simulink model "Modell_Aufzug"  (Simulink 8.5)
settings: Solver=ode45  StartTime=0.0  StopTime=Inf  MaxStep=step_max  RelTol=1e-3
values from neighbouring files (symbols this model uses):
  CE = 1.528    [Initdatei.m]
  CM = 1.528    [Initdatei.m]
  hsp = 1    [Initdatei.m]
  J = 0.012    [Initdatei.m]
  Kpi = LA/(2*(Tt+Tgl))    (= 1.81818181818)    [Initdatei.m]
  Kpn = (2*pi*J)/(CM*4*(Tt+Tgl))    (= 11.2146334612)    [Initdatei.m]
  Kpx = 1/(2*8*(Tt+Tgl)*hsp)    (= 56.8181818182)    [Initdatei.m]
  MLast = 10    [Initdatei.m]
  RA = 0.250    (= 0.25)    [Initdatei.m]
  TA = LA/RA    (= 0.016)    [Initdatei.m]
  Tgl = 0.001    [Initdatei.m]
  TN = 8*(Tt+Tgl)    (= 0.0088)    [Initdatei.m]
  Tt = 0.0001    [Initdatei.m]
  xSwitch_1_m = 4.50    (= 4.5)    [Initdatei.m]
  xSwitch_1_o = 5.50    (= 5.5)    [Initdatei.m]
  xSwitch_1_u = 3.50    (= 3.5)    [Initdatei.m]
  xSwitch_2_o = 9.0    (= 9)    [Initdatei.m]
  xSwitch_2_u = 8.00    (= 8)    [Initdatei.m]
  xSwitch_EG_o = 1    [Initdatei.m]
  xSwitch_EG_u = 0.20    (= 0.2)    [Initdatei.m]
libraries: simulink x6
settings Model: Creator=Fabian Horst  LastModifiedBy=thomas.stetz
settings DataIOCC: LimitDataPoints=off
settings DebuggingCC: SolverPrmCheckMsg=warning  FcnCallInpInsideContextMsg=UseLocalSettings

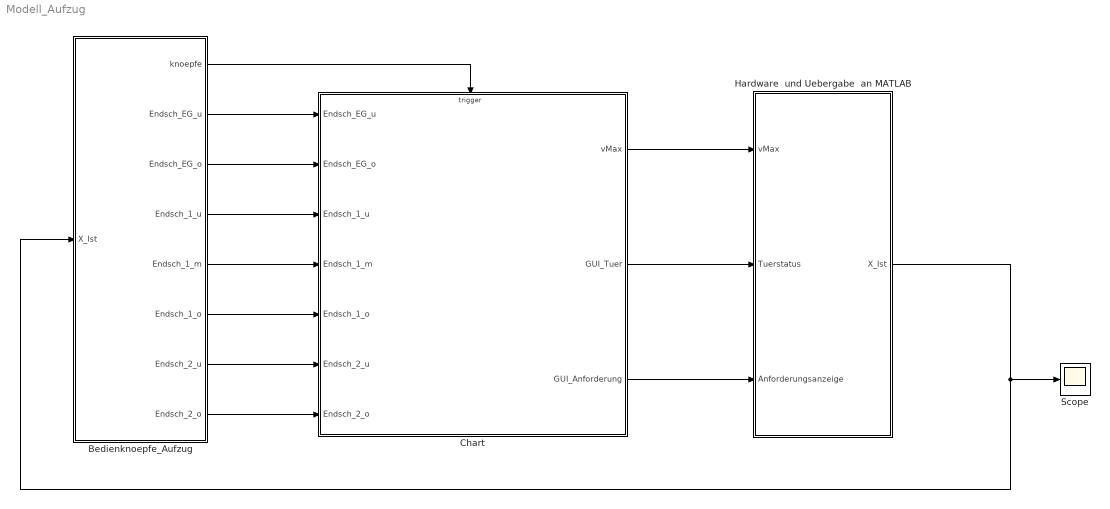
== system Modell_Aufzug ==
  Bedienknoepfe_Aufzug : Subsystem
  Chart : Stateflow chart  TreatAsAtomicUnit=on
  Hardware  und Uebergabe  an MATLAB : Subsystem
  Scope : Scope
  wires:
  Bedienknoepfe_Aufzug/1(knoepfe) -> Chart/Trigger
  Chart/1(vMax) -> Hardware  und Uebergabe  an MATLAB/1(vMax)
  Bedienknoepfe_Aufzug/8(Endsch_2_o) -> Chart/7(Endsch_2_o)
  Bedienknoepfe_Aufzug/2(Endsch_EG_u) -> Chart/1(Endsch_EG_u)
  Bedienknoepfe_Aufzug/3(Endsch_EG_o) -> Chart/2(Endsch_EG_o)
  Bedienknoepfe_Aufzug/4(Endsch_1_u) -> Chart/3(Endsch_1_u)
  Bedienknoepfe_Aufzug/6(Endsch_1_o) -> Chart/5(Endsch_1_o)
  Bedienknoepfe_Aufzug/7(Endsch_2_u) -> Chart/6(Endsch_2_u)
  Chart/2(GUI_Tuer) -> Hardware  und Uebergabe  an MATLAB/2(Tuerstatus)
  Hardware  und Uebergabe  an MATLAB/1(X_Ist) -> Bedienknoepfe_Aufzug/1(X_Ist), Scope/1
  Chart/3(GUI_Anforderung) -> Hardware  und Uebergabe  an MATLAB/3(Anforderungsanzeige)
  Bedienknoepfe_Aufzug/5(Endsch_1_m) -> Chart/4(Endsch_1_m)

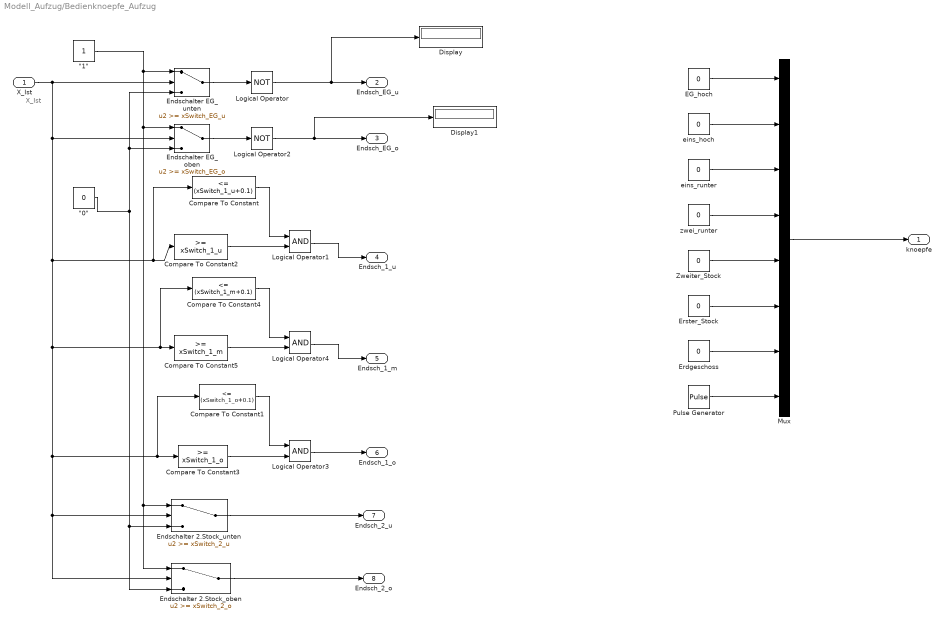
== system Modell_Aufzug/Bedienknoepfe_Aufzug ==
  note: X_Ist
  X_Ist : Inport  Description=X_Ist
  "\"0\"" : Constant  Value=0  OutDataTypeStr=boolean
  "\"1\"" : Constant  OutDataTypeStr=boolean
  Compare To Constant : simulink/Logic and Bit Operations/Compare To Constant  relop=<=  const=(xSwitch_1_u+0.1)  OutDataTypeStr=boolean
  Compare To Constant1 : simulink/Logic and Bit Operations/Compare To Constant  relop=<=  const=(xSwitch_1_o+0.1)  OutDataTypeStr=boolean
  Compare To Constant2 : simulink/Logic and Bit Operations/Compare To Constant  relop=>=  const=xSwitch_1_u  OutDataTypeStr=boolean
  Compare To Constant3 : simulink/Logic and Bit Operations/Compare To Constant  relop=>=  const=xSwitch_1_o  OutDataTypeStr=boolean
  Compare To Constant4 : simulink/Logic and Bit Operations/Compare To Constant  relop=<=  const=(xSwitch_1_m+0.1)  OutDataTypeStr=boolean
  Compare To Constant5 : simulink/Logic and Bit Operations/Compare To Constant  relop=>=  const=xSwitch_1_m  OutDataTypeStr=boolean
  Display : Display
  Display1 : Display
  EG_hoch : Constant  Value=0
  Endschalter 2.Stock_oben : Switch  Threshold=xSwitch_2_o
  Endschalter 2.Stock_unten : Switch  Threshold=xSwitch_2_u
  Endschalter EG_oben : Switch  Threshold=xSwitch_EG_o
  Endschalter EG_unten : Switch  Threshold=xSwitch_EG_u
  Erdgeschoss : Constant  Value=0
  Erster_Stock : Constant  Value=0
  Logical Operator : Logic  Operator=NOT  AllPortsSameDT=off  OutDataTypeStr=boolean
  Logical Operator1 : Logic  AllPortsSameDT=off  OutDataTypeStr=boolean
  Logical Operator2 : Logic  Operator=NOT  AllPortsSameDT=off  OutDataTypeStr=boolean
  Logical Operator3 : Logic  AllPortsSameDT=off  OutDataTypeStr=boolean
  Logical Operator4 : Logic  AllPortsSameDT=off  OutDataTypeStr=boolean
  Mux : Mux  Inputs=8
  Pulse Generator : DiscretePulseGenerator  PulseType=Time based  Period=0.001  PulseWidth=50
  Zweiter_Stock : Constant  Value=0
  eins_hoch : Constant  Value=0
  eins_runter : Constant  Value=0
  zwei_runter : Constant  Value=0
  knoepfe : Outport
  Endsch_EG_u : Outport  Port=2
  Endsch_EG_o : Outport  Port=3
  Endsch_1_u : Outport  Port=4
  Endsch_1_m : Outport  Port=5
  Endsch_1_o : Outport  Port=6
  Endsch_2_u : Outport  Port=7
  Endsch_2_o : Outport  Port=8
  wires:
  EG_hoch/1 -> Mux/1
  eins_hoch/1 -> Mux/2
  eins_runter/1 -> Mux/3
  zwei_runter/1 -> Mux/4
  Zweiter_Stock/1 -> Mux/5
  Erdgeschoss/1 -> Mux/7
  Mux/1 -> knoepfe/1
  "\"1\""/1 -> Endschalter EG_unten/1, Endschalter EG_oben/1, Endschalter 2.Stock_unten/1, Endschalter 2.Stock_oben/1
  "\"0\""/1 -> Endschalter EG_unten/3, Endschalter EG_oben/3, Endschalter 2.Stock_unten/3, Endschalter 2.Stock_oben/3
  X_Ist/1 -> Endschalter EG_unten/2, Compare To Constant/1, Compare To Constant2/1, Compare To Constant1/1, Compare To Constant3/1, Endschalter 2.Stock_oben/2, Endschalter 2.Stock_unten/2, Compare To Constant5/1, Compare To Constant4/1, Endschalter EG_oben/2
  Endschalter 2.Stock_unten/1 -> Endsch_2_u/1
  Erster_Stock/1 -> Mux/6
  Endschalter EG_unten/1 -> Logical Operator/1
  Logical Operator/1 -> Endsch_EG_u/1, Display/1
  Logical Operator1/1 -> Endsch_1_u/1
  Compare To Constant/1 -> Logical Operator1/1
  Compare To Constant2/1 -> Logical Operator1/2
  Pulse Generator/1 -> Mux/8
  Endschalter EG_oben/1 -> Logical Operator2/1
  Logical Operator2/1 -> Endsch_EG_o/1, Display1/1
  Logical Operator3/1 -> Endsch_1_o/1
  Compare To Constant1/1 -> Logical Operator3/1
  Compare To Constant3/1 -> Logical Operator3/2
  Endschalter 2.Stock_oben/1 -> Endsch_2_o/1
  Logical Operator4/1 -> Endsch_1_m/1
  Compare To Constant4/1 -> Logical Operator4/1
  Compare To Constant5/1 -> Logical Operator4/2

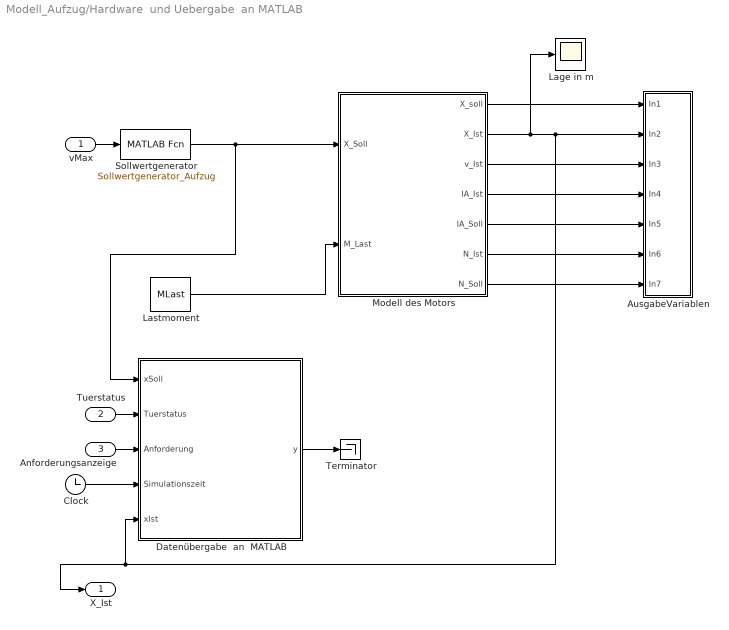
== system Modell_Aufzug/Hardware  und Uebergabe  an MATLAB ==
  vMax : Inport
  Tuerstatus : Inport  Port=2
  Anforderungsanzeige : Inport  Port=3
  AusgabeVariablen : Subsystem
  Clock : Clock
  Datenübergabe  an  MATLAB : MATLAB Function  TreatAsAtomicUnit=on
  Lage in m : Scope
      settings: TimeRange=20  YMin=-1  YMax=14
  Lastmoment : Constant  Value=MLast
  Modell des Motors : Subsystem
  Sollwertgenerator : MATLABFcn  MATLABFcn=Sollwertgenerator_Aufzug
  Terminator : Terminator
  X_Ist : Outport
  wires:
  Modell des Motors/1(X_soll) -> AusgabeVariablen/1(In1)
  Modell des Motors/2(X_Ist) -> AusgabeVariablen/2(In2), Datenübergabe  an  MATLAB/5(xIst), X_Ist/1, Lage in m/1
  Modell des Motors/3(v_Ist) -> AusgabeVariablen/3(In3)
  Modell des Motors/4(IA_Ist) -> AusgabeVariablen/4(In4)
  Modell des Motors/5(IA_Soll) -> AusgabeVariablen/5(In5)
  Modell des Motors/6(N_Ist) -> AusgabeVariablen/6(In6)
  Modell des Motors/7(N_Soll) -> AusgabeVariablen/7(In7)
  Lastmoment/1 -> Modell des Motors/2(M_Last)
  Clock/1 -> Datenübergabe  an  MATLAB/4(Simulationszeit)
  Sollwertgenerator/1 -> Datenübergabe  an  MATLAB/1(xSoll), Modell des Motors/1(X_Soll)
  vMax/1 -> Sollwertgenerator/1
  Tuerstatus/1 -> Datenübergabe  an  MATLAB/2(Tuerstatus)
  Datenübergabe  an  MATLAB/1(y) -> Terminator/1
  Anforderungsanzeige/1 -> Datenübergabe  an  MATLAB/3(Anforderung)

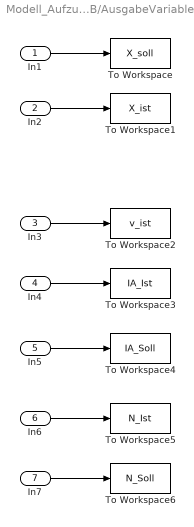
== system Modell_Aufzug/Hardware  und Uebergabe  an MATLAB/AusgabeVariablen ==
  In1 : Inport
  In2 : Inport  Port=2
  In3 : Inport  Port=3
  In4 : Inport  Port=4
  In5 : Inport  Port=5
  In6 : Inport  Port=6
  In7 : Inport  Port=7
  To Workspace : ToWorkspace  VariableName=X_soll  SaveFormat=Structure  SampleTime=-1
  To Workspace1 : ToWorkspace  VariableName=X_ist  SaveFormat=Structure  SampleTime=-1
  To Workspace2 : ToWorkspace  VariableName=v_ist  SaveFormat=Structure  SampleTime=-1
  To Workspace3 : ToWorkspace  VariableName=IA_Ist  SaveFormat=Structure  SampleTime=-1
  To Workspace4 : ToWorkspace  VariableName=IA_Soll  SaveFormat=Structure  SampleTime=-1
  To Workspace5 : ToWorkspace  VariableName=N_Ist  SaveFormat=Structure  SampleTime=-1
  To Workspace6 : ToWorkspace  VariableName=N_Soll  SaveFormat=Structure  SampleTime=-1
  wires:
  In1/1 -> To Workspace/1
  In2/1 -> To Workspace1/1
  In3/1 -> To Workspace2/1
  In4/1 -> To Workspace3/1
  In5/1 -> To Workspace4/1
  In6/1 -> To Workspace5/1
  In7/1 -> To Workspace6/1

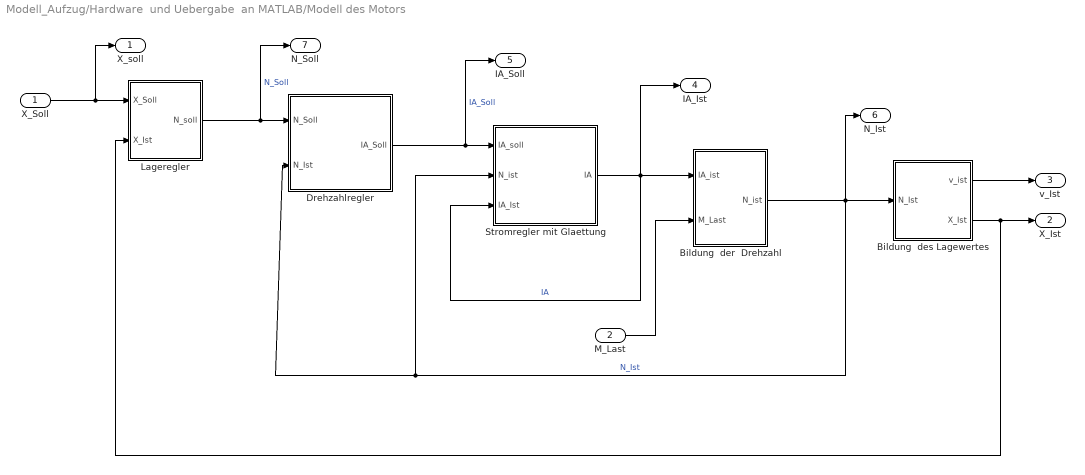
== system Modell_Aufzug/Hardware  und Uebergabe  an MATLAB/Modell des Motors ==
  X_Soll : Inport
  M_Last : Inport  Port=2
  Bildung  der  Drehzahl : Subsystem
  Bildung  des Lagewertes : Subsystem
  Drehzahlregler : Subsystem
  Lageregler : Subsystem
  Stromregler mit Glaettung : Subsystem
  X_soll : Outport
  X_Ist : Outport  Port=2
  v_Ist : Outport  Port=3
  IA_Ist : Outport  Port=4
  IA_Soll : Outport  Port=5
  N_Ist : Outport  Port=6
  N_Soll : Outport  Port=7
  wires:
  Lageregler/1(N_soll) -> Drehzahlregler/1(N_Soll), N_Soll/1  "N_Soll"
  Drehzahlregler/1(IA_Soll) -> Stromregler mit Glaettung/1(IA_soll), IA_Soll/1  "IA_Soll"
  X_Soll/1 -> Lageregler/1(X_Soll), X_soll/1
  Stromregler mit Glaettung/1(IA) -> Bildung  der  Drehzahl/1(IA_ist), Stromregler mit Glaettung/3(IA_Ist), IA_Ist/1  "IA"
  Bildung  der  Drehzahl/1(N_ist) -> Bildung  des Lagewertes/1(N_Ist), Drehzahlregler/2(N_Ist), Stromregler mit Glaettung/2(N_ist), N_Ist/1  "N_Ist"
  M_Last/1 -> Bildung  der  Drehzahl/2(M_Last)
  Bildung  des Lagewertes/1(v_ist) -> v_Ist/1
  Bildung  des Lagewertes/2(X_Ist) -> X_Ist/1, Lageregler/2(X_Ist)

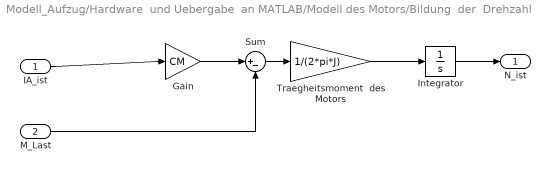
== system Modell_Aufzug/Hardware  und Uebergabe  an MATLAB/Modell des Motors/Bildung  der  Drehzahl ==
  IA_ist : Inport
  M_Last : Inport  Port=2
  Gain : Gain  Gain=CM
  Integrator : Integrator
  Sum : Sum  Inputs=|+-
  Traegheitsmoment  des Motors : Gain  Gain=1/(2*pi*J)
  N_ist : Outport
  wires:
  IA_ist/1 -> Gain/1
  M_Last/1 -> Sum/2
  Gain/1 -> Sum/1
  Sum/1 -> Traegheitsmoment  des Motors/1
  Traegheitsmoment  des Motors/1 -> Integrator/1
  Integrator/1 -> N_ist/1

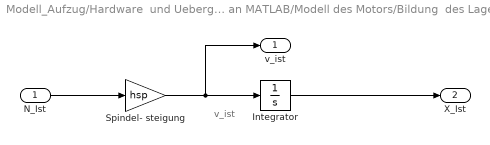
== system Modell_Aufzug/Hardware  und Uebergabe  an MATLAB/Modell des Motors/Bildung  des Lagewertes ==
  note: v_ist
  N_Ist : Inport
  Integrator : Integrator
  Spindel- steigung : Gain  Gain=hsp
  v_ist : Outport
  X_Ist : Outport  Port=2
  wires:
  N_Ist/1 -> Spindel- steigung/1
  Spindel- steigung/1 -> Integrator/1, v_ist/1
  Integrator/1 -> X_Ist/1

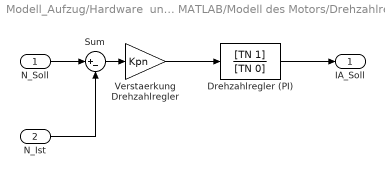
== system Modell_Aufzug/Hardware  und Uebergabe  an MATLAB/Modell des Motors/Drehzahlregler ==
  N_Soll : Inport
  N_Ist : Inport  Port=2
  Drehzahlregler (PI) : TransferFcn  Numerator=[TN 1]  Denominator=[TN 0]
  Sum : Sum  Inputs=|+-
  Verstaerkung Drehzahlregler : Gain  Gain=Kpn
  IA_Soll : Outport
  wires:
  N_Ist/1 -> Sum/2
  N_Soll/1 -> Sum/1
  Sum/1 -> Verstaerkung Drehzahlregler/1
  Drehzahlregler (PI)/1 -> IA_Soll/1
  Verstaerkung Drehzahlregler/1 -> Drehzahlregler (PI)/1

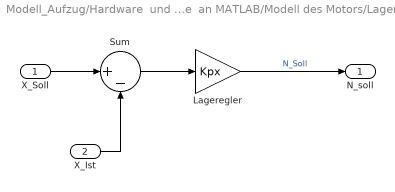
== system Modell_Aufzug/Hardware  und Uebergabe  an MATLAB/Modell des Motors/Lageregler ==
  X_Soll : Inport
  X_Ist : Inport  Port=2
  Lageregler : Gain  Gain=Kpx
  Sum : Sum  Inputs=|+-
  N_soll : Outport
  wires:
  X_Soll/1 -> Sum/1
  Sum/1 -> Lageregler/1
  Lageregler/1 -> N_soll/1  "N_Soll"
  X_Ist/1 -> Sum/2

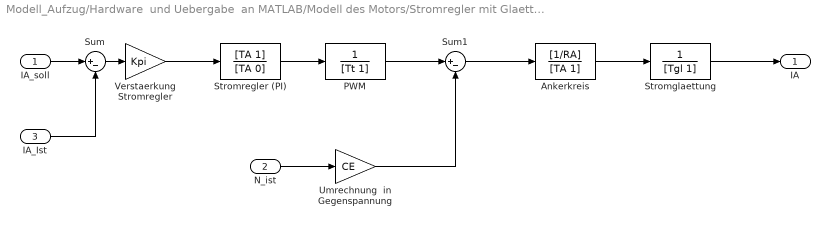
== system Modell_Aufzug/Hardware  und Uebergabe  an MATLAB/Modell des Motors/Stromregler mit Glaettung ==
  IA_soll : Inport
  N_ist : Inport  Port=2
  IA_Ist : Inport  Port=3
  Ankerkreis : TransferFcn  Numerator=[1/RA]  Denominator=[TA 1]
  PWM : TransferFcn  Denominator=[Tt 1]
  Stromglaettung : TransferFcn  Denominator=[Tgl 1]
  Stromregler (PI) : TransferFcn  Numerator=[TA 1]  Denominator=[TA 0]
  Sum : Sum  Inputs=|+-
  Sum1 : Sum  Inputs=|+-
  Umrechnung  in Gegenspannung : Gain  Gain=CE
  Verstaerkung Stromregler : Gain  Gain=Kpi
  IA : Outport
  wires:
  IA_Ist/1 -> Sum/2
  IA_soll/1 -> Sum/1
  Sum/1 -> Verstaerkung Stromregler/1
  Verstaerkung Stromregler/1 -> Stromregler (PI)/1
  Stromregler (PI)/1 -> PWM/1
  PWM/1 -> Sum1/1
  N_ist/1 -> Umrechnung  in Gegenspannung/1
  Umrechnung  in Gegenspannung/1 -> Sum1/2
  Sum1/1 -> Ankerkreis/1
  Ankerkreis/1 -> Stromglaettung/1
  Stromglaettung/1 -> IA/1

== stateflow chart Chart ==
  settings: executeAtInitialization=1
  state Steuerung
    state Anforderungen [parallel]
      settings: executionOrder=1
      state Anf_Stock2_innen/
        en: anf_2 = 1;
        en: GUI_Anforderung = 7;
      state Anf_1_runter_aussen/
        en: anf_1_runter = 1;
        en: GUI_Anforderung = 5;
      state Anf_1_hoch_innen/
        en: anf_1_hoch = 1;
        en: anf_1_runter = 1;
        en: GUI_Anforderung = 4;
      state Anf_1_hoch_aussen/
        en: anf_1_hoch = 1;
        en: GUI_Anforderung = 3;
      state Anf_EG_aussen/
        en: anf_EG = 1;
        en: GUI_Anforderung = 1;
      state Warte
      state Anf_Stock2_aussen/
        en: anf_2 = 1;
        en: GUI_Anforderung = 6;
      state Anf_EG1_innen/
        en: anf_EG = 1;
        en: GUI_Anforderung = 2;
      (default) -> Warte
      (junction 28) -> Warte
      Warte -> (junction 29)
      (junction 29) -> Anf_EG_aussen [order 1] : S0_0
      Anf_EG_aussen -> (junction 28)
      Anf_EG1_innen -> (junction 28)
      (junction 29) -> Anf_EG1_innen [order 7] : S3_0
      Anf_1_hoch_aussen -> (junction 28)
      Anf_1_hoch_innen -> (junction 28)
      Anf_1_runter_aussen -> (junction 28)
      Anf_Stock2_innen -> (junction 28)
      Anf_Stock2_aussen -> (junction 28)
      (junction 29) -> Anf_1_hoch_aussen [order 2] : S1_0
      (junction 29) -> Anf_1_hoch_innen [order 3] : S3_1
      (junction 29) -> Anf_1_runter_aussen [order 4] : S1_1
      (junction 29) -> Anf_Stock2_aussen [order 6] : S2_0
      (junction 29) -> Anf_Stock2_innen [order 5] : S3_2
    state Steuerung_Aufzug [parallel]
      settings: executionOrder=2
      state EG
        state Bremsen/
          en: vMax = -0.5;
        state Tuer_zu/
          en: vMax = 0;
          en: GUI_Tuer = 4; %für GUI
        state Tuer_geoffnet/
          en: GUI_Tuer = 0;
          en: anf_EG = 0;
        state Tuer_oeffnet/
          en: GUI_Tuer = 0.5;
        state Tuer_schliesst/
          en: GUI_Tuer = 0.5;
        Steuerung.Steuerung_Aufzug.EG.Tuer_zu -> Steuerung.Steuerung_Aufzug.EG.Tuer_oeffnet [order 2] : after(500,TIMER)
        Steuerung.Steuerung_Aufzug.EG.Tuer_oeffnet -> Tuer_geoffnet : after(500,TIMER)
        (default) -> Steuerung.Steuerung_Aufzug.EG.Tuer_zu
        Steuerung.Steuerung_Aufzug.EG.Bremsen -> Steuerung.Steuerung_Aufzug.EG.Tuer_zu : [Endsch_EG_u==1]
        Steuerung.Steuerung_Aufzug.EG.Tuer_schliesst -> Steuerung.Steuerung_Aufzug.EG.Tuer_zu : after(500,TIMER)
        Tuer_geoffnet -> Steuerung.Steuerung_Aufzug.EG.Tuer_schliesst : after(500,TIMER)
      state Stock_2
        state Bremsen/
          en: vMax = 0.5;
        state Tuer_zu/
          en: vMax = 0;
          en: GUI_Tuer = 4; %für GUI
        state Tuer_oeffnet/
          en: GUI_Tuer = 2.5;
        state Tuer_schliesst/
          en: GUI_Tuer = 2.5;
        state Tuer_geoeffnet/
          en: GUI_Tuer = 2;
          en: anf_2 = 0;
        Steuerung.Steuerung_Aufzug.Stock_2.Bremsen -> Steuerung.Steuerung_Aufzug.Stock_2.Tuer_zu : [Endsch_2_o==1]
        Steuerung.Steuerung_Aufzug.Stock_2.Tuer_zu -> Steuerung.Steuerung_Aufzug.Stock_2.Tuer_oeffnet [order 2] : after(500,TIMER)
        Steuerung.Steuerung_Aufzug.Stock_2.Tuer_oeffnet -> Tuer_geoeffnet : after(500,TIMER)
        (default) -> Steuerung.Steuerung_Aufzug.Stock_2.Tuer_zu
        Steuerung.Steuerung_Aufzug.Stock_2.Tuer_schliesst -> Steuerung.Steuerung_Aufzug.Stock_2.Tuer_zu : after(500,TIMER)
        Tuer_geoeffnet -> Steuerung.Steuerung_Aufzug.Stock_2.Tuer_schliesst : after(500,TIMER)
      state nach_oben/
        en: vMax = 4;
      state nach_unten/
        en: vMax = -4;
      Steuerung.Steuerung_Aufzug.EG.Tuer_zu -> nach_oben [order 1] : [anf_2 == 1]
      nach_oben -> Steuerung.Steuerung_Aufzug.Stock_2.Bremsen : [anf_2==1&&Endsch_2_u==1]
      Steuerung.Steuerung_Aufzug.Stock_2.Tuer_zu -> nach_unten [order 1] : [anf_EG==1]
      nach_unten -> Steuerung.Steuerung_Aufzug.EG.Bremsen : [anf_EG==1&&Endsch_EG_o==1]
      (default) -> EG
  data: vMax output double; anf_EG local boolean; anf_1_hoch local boolean; anf_1_runter local boolean; anf_2 local boolean; Endsch_EG_u input boolean; Endsch_EG_o input boolean; Endsch_1_u input boolean; Endsch_1_m input boolean; Endsch_1_o input boolean; Endsch_2_u input boolean; Endsch_2_o input boolean; GUI_Tuer output double; GUI_Anforderung output double
  data anf_EG settings: description=Anforderung Erdgeschoss nach oben
  data anf_1_hoch settings: description=Anforderung 1.Stock nach oben
  data anf_1_runter settings: description=Anforderung 1.Stock nach unten
  data anf_2 settings: description=Anforderung 2. Stock nach unten
  data GUI_Anforderung settings: description=Ausgang zur Übergabe an MATLAB
  events: S0_0 input RISING_EDGE_EVENT; S1_0 input RISING_EDGE_EVENT; S1_1 input RISING_EDGE_EVENT; S2_0 input RISING_EDGE_EVENT; S3_2 input RISING_EDGE_EVENT; S3_1 input RISING_EDGE_EVENT; S3_0 input RISING_EDGE_EVENT; TIMER input EITHER_EDGE_EVENT

== matlab function Hardware und Uebergabe an MATLAB/Datenübergabe an MATLAB ==
  data: xSoll input double; Tuerstatus input double; Anforderung input double; y output double; Simulationszeit input double; xIst input double
function y = fcn(xSoll,Tuerstatus,Anforderung,Simulationszeit,xIst)
%Funktion zum Uebergeben der Simulationszeit und X-Sollwert an MATLAB

eml.extrinsic('assignin')                                                   %Laedt die Funktion 'assignin' aus der Bibliothek  
assignin('base','tsim',Simulationszeit);                                    %Schreibt die aktuelle Simulationszeit in 'tsim'
assignin('base','GUI_Tuer',Tuerstatus);                                  %Schreibt den Status der Tuer in 'Tuer_Status'
assignin('base','xSoll',xSoll);                                     %schreibt die aktuelle Position in 'XSollwert'
assignin('base','GUI_xIst',xIst);                                         %schreibt die aktuelle Position in 'X_aktuell'
assignin('base','GUI_Anforderung',Anforderung);                                %schreibt die aktuelle Stockwerksanforderung in 'Anforderung'

y=0;                                                                        %Ausgang hiervon wird nicht benoetigt-> auf Terminator
